simulink model "cart_pend_to_workspace"  (R2019b)
settings: Solver=FixedStepAuto  StartTime=0.0  StopTime=100  FixedStep=0.01  RelTol=1e-3
settings Model: Creator=Murray  LastModifiedBy=Murray

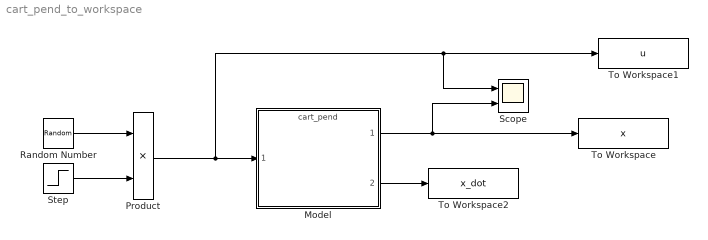
== system cart_pend_to_workspace ==
  Model : ModelReference  ModelNameDialog=cart_pend  SimulationMode=Normal  ModelReferenceVersion=1.19
  Product : Product
  Random Number : RandomNumber  Variance=5  SampleTime=2
  Scope : Scope  NumInputPorts=2
  Step : Step  Before=1  SampleTime=0
  To Workspace : ToWorkspace  VariableName=x  SaveFormat=Timeseries  SampleTime=-1
  To Workspace1 : ToWorkspace  VariableName=u  SaveFormat=Timeseries  SampleTime=-1
  To Workspace2 : ToWorkspace  VariableName=x_dot  SaveFormat=Timeseries  SampleTime=-1
  wires:
  Product/1 -> Scope/1, To Workspace1/1, Model/1
  Model/1 -> Scope/2, To Workspace/1
  Model/2 -> To Workspace2/1
  Random Number/1 -> Product/1
  Step/1 -> Product/2
